simulink model "AuE6610_Project_EV"  (R2025a)
settings: Solver=FixedStepAuto  StartTime=0.0  StopTime=3353  FixedStep=1  RelTol=1e-3
values from neighbouring files (symbols this model uses):
  area_frontal = 2.18    [CV_Powertrain.m]    (also in EV_Powertrain.m; database.m)
  batt =     [battery_data.mat]
  curb_weight = 1377    [CV_Powertrain.m]    (also in EV_Powertrain.m; database.m)
  drag_coefficient = 0.29    [CV_Powertrain.m]    (also in EV_Powertrain.m; database.m)
  fdr = 4.21    [CV_Powertrain.m]    (also in EV_Powertrain.m; database.m)
  fdr_inertia = 0.02    [CV_Powertrain.m]    (also in EV_Powertrain.m; database.m)
  gear = [3.54, 1.91, 1.31, 0.97, 0.71, 0.62]    [CV_Powertrain.m]    (also in EV_Powertrain.m = 1.5; database.m)
  gear_no = [1, 2, 3, 4, 5, 6]    [CV_Powertrain.m]    (also in EV_Powertrain.m = 1; database.m = [1,2,3,4,5,6])
  mot =     [motor_data.mat]
  radius = 0.4318    [CV_Powertrain.m]    (also in EV_Powertrain.m; database.m)
  rho_air = 1.18    [CV_Powertrain.m]    (also in EV_Powertrain.m = 1.21; database.m)
  rolling_resistance_coefficient = 0.01    [CV_Powertrain.m]    (also in EV_Powertrain.m; database.m)
  trans_inertia = 0.04    [CV_Powertrain.m]    (also in EV_Powertrain.m; database.m)
  wheel_inertia = 0.95    [CV_Powertrain.m]    (also in EV_Powertrain.m; database.m)
libraries: slpidlib x2, simulink x2
settings Model: Creator=Qilun Zhu  LastModifiedBy=abhi
settings SolverCC: ZeroCrossAlgorithm=Adaptive  AlgebraicLoopSolver=TrustRegion
settings DataIOCC: ReturnWorkspaceOutputs=off
settings DebuggingCC: UnconnectedInputMsg=warning  UnconnectedOutputMsg=warning  UnconnectedLineMsg=warning  ArithmeticOperatorsInVariantConditions=warning
settings ModelReferenceCC: EnableRefExpFcnMdlSchedulingChecks=on
settings SFSimCC: SimUseLocalCustomCode=off  CustomCodeUndefinedFunction=UseInterfaceOnly
settings RTWCC: RTWUseLocalCustomCode=off  GPUComputeCapability=3.5  DLArmComputeVersion=19.05
settings CodeAppCC: StateflowObjectComments=on
settings SimscapeCC: SimscapeNormalizeSystem=off

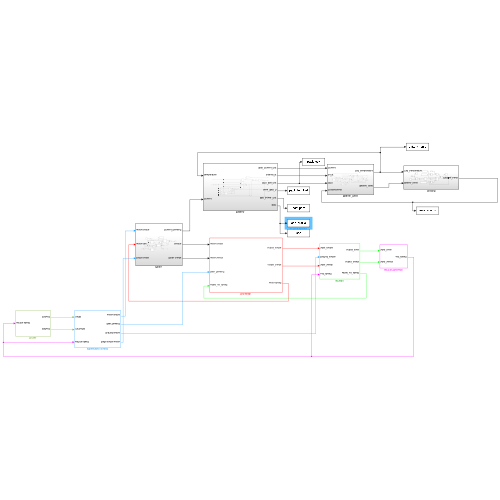
[thumbnail: Simulink's stored preview of the top-level diagram]
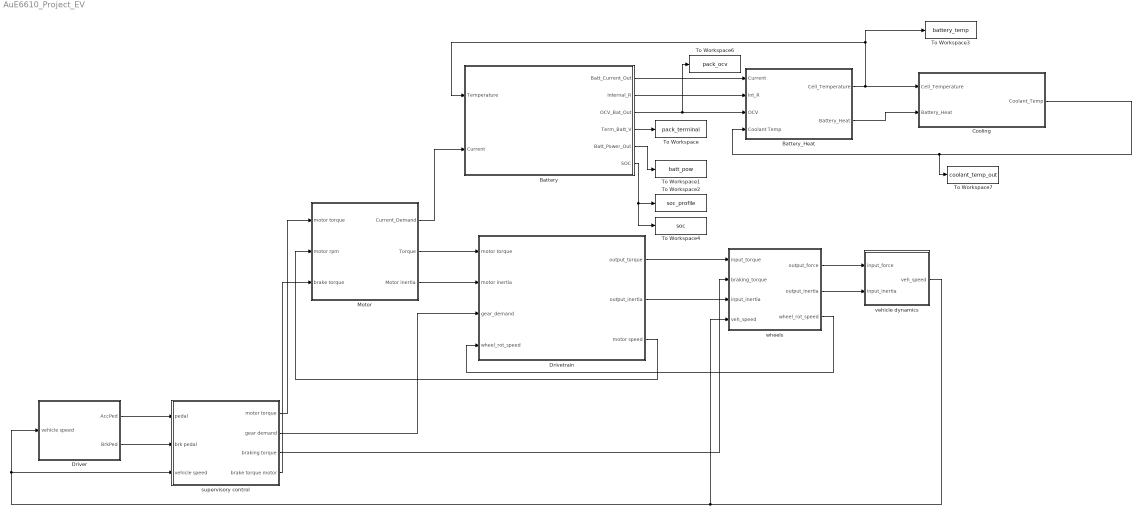
== system AuE6610_Project_EV ==
  Battery : Subsystem
  Battery_Heat : Subsystem
  Cooling : Subsystem
  Driver : Subsystem
  Drivetrain : Subsystem
  Motor : Subsystem
  To Workspace : ToWorkspace  VariableName=pack_terminal  SampleTime=-1
  To Workspace1 : ToWorkspace  VariableName=batt_pow  SampleTime=-1
  To Workspace2 : ToWorkspace  VariableName=soc_profile  SampleTime=300
  To Workspace3 : ToWorkspace  VariableName=battery_temp  SampleTime=-1
  To Workspace4 : ToWorkspace  VariableName=soc  SampleTime=-1
  To Workspace6 : ToWorkspace  VariableName=pack_ocv  SampleTime=-1
  To Workspace7 : ToWorkspace  VariableName=coolant_temp_out  SampleTime=-1
  supervisory control : Subsystem
  vehicle dynamics : Subsystem
  wheels : Subsystem
  wires:
  supervisory control/1(motor torque) -> Motor/1(motor torque)
  wheels/1(output_force) -> vehicle dynamics/1(input_force)
  wheels/2(output_inertia) -> vehicle dynamics/2(input_inertia)
  supervisory control/3(braking torque) -> wheels/2(braking_torque)
  Driver/1(AccPed) -> supervisory control/1(" pedal")
  supervisory control/2(gear demand) -> Drivetrain/3(gear_demand)
  Motor/2(Torque) -> Drivetrain/1(motor torque)
  Motor/3(Motor inertia) -> Drivetrain/2(motor inertia)
  wheels/3(wheel_rot_speed) -> Drivetrain/4(wheel_rot_speed)
  Drivetrain/1(output_torque) -> wheels/1(input_torque)
  Drivetrain/2(output_inertia) -> wheels/3(input_inertia)
  vehicle dynamics/1(veh_speed) -> Driver/1(vehicle speed), supervisory control/3(vehicle speed), wheels/4(veh_speed)
  Driver/2(BrkPed) -> supervisory control/2(" brk pedal")
  Motor/1(Current_Demand) -> Battery/2(Current)
  Battery_Heat/1(Cell_Temperature) -> Cooling/1(Cell_Temperature), To Workspace3/1, Battery/1(Temperature)
  Battery_Heat/2(Battery_Heat) -> Cooling/2(Battery_Heat)
  Cooling/1(Coolant_Temp) -> To Workspace7/1, Battery_Heat/4(Coolant Temp)
  Battery/3(OCV_Bat_Out) -> To Workspace6/1, Battery_Heat/3(OCV)
  Battery/2(Internal_R) -> Battery_Heat/2(Int_R)
  Battery/1(Batt_Current_Out) -> Battery_Heat/1(Current)
  Battery/4(Term_Batt_V) -> To Workspace/1
  Battery/5(Batt_Power_Out) -> To Workspace1/1
  Battery/6(SOC) -> To Workspace4/1, To Workspace2/1
  Drivetrain/3(motor speed) -> Motor/2(motor rpm)
  supervisory control/4(brake torque motor) -> Motor/3(brake torque)

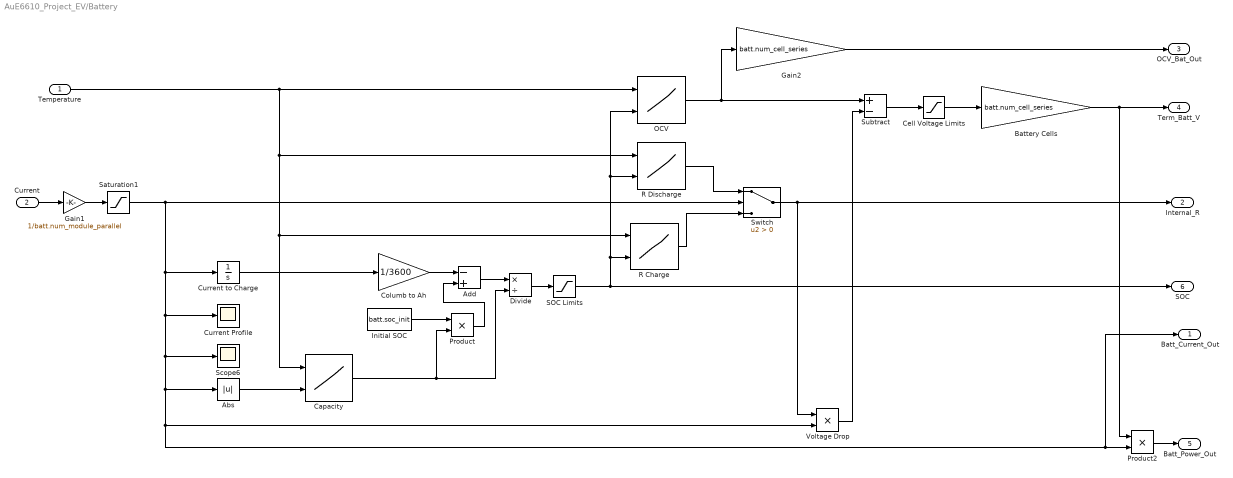
== system AuE6610_Project_EV/Battery ==
  Temperature : Inport
  Current : Inport  Port=2
  Abs : Abs  SaturateOnIntegerOverflow=off
  Add : Sum  Inputs=-+
  Battery Cells : Gain  Gain=batt.num_cell_series
  Capacity : Lookup_n-D  BreakpointsForDimension1=batt.cap_max.temp  BreakpointsForDimension2=batt.cap_max.curr  Table=batt.cap_max.cap_max  InternalRulePriority=Speed  RndMeth=Simplest
      settings: InputPortMap=u0,u1
  Cell Voltage Limits : Saturate  UpperLimit=batt.volt_max  LowerLimit=batt.volt_min
  Columb to Ah : Gain  Gain=1/3600
  Current Profile : Scope
      settings: ActiveDisplayYMinimum=-1  ActiveDisplayYMaximum=1
  Current to Charge : Integrator
  Divide : Product  Inputs=*/
  Gain1 : Gain  Gain=1/batt.num_module_parallel
  Gain2 : Gain  Gain=batt.num_cell_series
  Initial SOC : Constant  Value=batt.soc_init
  OCV : Lookup_n-D  BreakpointsForDimension1=batt.voc.temp  BreakpointsForDimension2=batt.voc.soc  Table=batt.voc.voc  InternalRulePriority=Speed  RndMeth=Simplest
      settings: InputPortMap=u0,u1
  Product : Product
  Product2 : Product
  R Charge : Lookup_n-D  BreakpointsForDimension1=batt.r_int_chg.temp  BreakpointsForDimension2=batt.r_int_chg.soc  Table=batt.r_int_chg.r_int  InternalRulePriority=Speed  RndMeth=Simplest
      settings: InputPortMap=u0,u1
  R Discharge : Lookup_n-D  BreakpointsForDimension1=batt.r_int_dis.temp  BreakpointsForDimension2=batt.r_int_dis.soc  Table=batt.r_int_dis.r_int  InternalRulePriority=Speed  RndMeth=Simplest
      settings: InputPortMap=u0,u1
  SOC Limits : Saturate  UpperLimit=batt.soc_max  LowerLimit=batt.soc_min
  Saturation1 : Saturate  UpperLimit=batt.curr_dis_max  LowerLimit=batt.curr_chg_max
  Scope6 : Scope
      settings: ActiveDisplayYMinimum=-1  ActiveDisplayYMaximum=1  DataLoggingVariableName=ScopeData7
  Subtract : Sum  Inputs=+-
  Switch : Switch  Criteria=u2 > Threshold  SaturateOnIntegerOverflow=off  InputSameDT=off
  Voltage Drop : Product
  Batt_Current_Out : Outport
  Internal_R : Outport  Port=2
  OCV_Bat_Out : Outport  Port=3
  Term_Batt_V : Outport  Port=4
  Batt_Power_Out : Outport  Port=5
  SOC : Outport  Port=6
  wires:
  Product2/1 -> Batt_Power_Out/1
  Subtract/1 -> Cell Voltage Limits/1
  Voltage Drop/1 -> Subtract/2
  Battery Cells/1 -> Term_Batt_V/1, Product2/1
  Gain2/1 -> OCV_Bat_Out/1
  R Charge/1 -> Switch/3
  R Discharge/1 -> Switch/1
  Temperature/1 -> Capacity/1, R Charge/1, R Discharge/1, OCV/1
  Divide/1 -> SOC Limits/1
  Add/1 -> Divide/1
  Cell Voltage Limits/1 -> Battery Cells/1
  Product/1 -> Add/2
  Switch/1 -> Internal_R/1, Voltage Drop/1
  Initial SOC/1 -> Product/1
  Abs/1 -> Capacity/2
  SOC Limits/1 -> R Charge/2, OCV/2, R Discharge/2, SOC/1
  Current/1 -> Gain1/1
  Current to Charge/1 -> Columb to Ah/1
  Columb to Ah/1 -> Add/1
  OCV/1 -> Gain2/1, Subtract/1
  Capacity/1 -> Product/2, Divide/2
  Saturation1/1 -> Batt_Current_Out/1, Product2/2, Voltage Drop/2, Abs/1, Scope6/1, Current Profile/1, Current to Charge/1, Switch/2
  Gain1/1 -> Saturation1/1

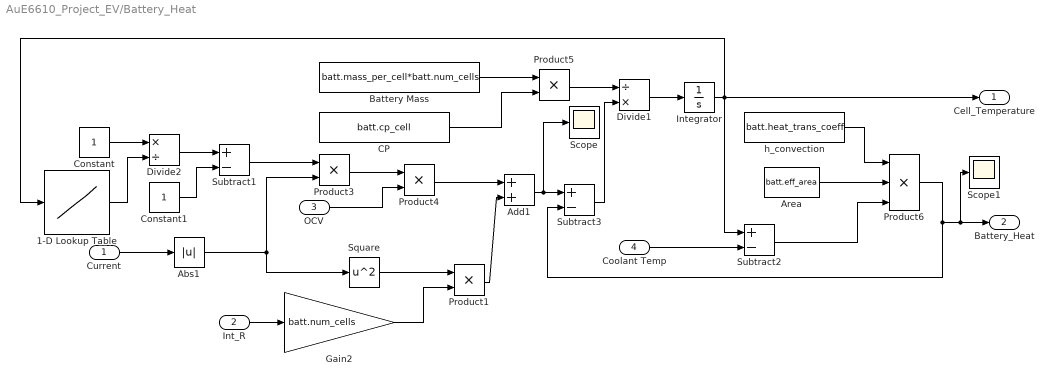
== system AuE6610_Project_EV/Battery_Heat ==
  Current : Inport
  Int_R : Inport  Port=2
  OCV : Inport  Port=3
  Coolant Temp : Inport  Port=4
  1-D Lookup Table : Lookup_n-D  NumberOfTableDimensions=1  BreakpointsForDimension1=batt.col_eff.temperature  Table=batt.col_eff.col_eff  InternalRulePriority=Speed  RndMeth=Simplest
  Abs1 : Abs  SaturateOnIntegerOverflow=off
  Add1 : Sum
  Area : Constant  Value=batt.eff_area
  Battery Mass : Constant  Value=batt.mass_per_cell*batt.num_cells
  CP : Constant  Value=batt.cp_cell
  Constant : Constant
  Constant1 : Constant
  Divide1 : Product  Inputs=/*
  Divide2 : Product  Inputs=*/
  Gain2 : Gain  Gain=batt.num_cells
  Integrator : Integrator  InitialCondition=25
  Product{1,3..5} (4 alike) : Product
  Product6 : Product  Inputs=3
  Scope : Scope
      settings: ActiveDisplayYMinimum=-1  ActiveDisplayYMaximum=1  DataLoggingVariableName=ScopeData2
  Scope1 : Scope
      settings: ActiveDisplayYMinimum=-470.32626460451758  ActiveDisplayYMaximum=4232.9363814406588  DataLoggingVariableName=ScopeData14
  Square : Math  Operator=square
  Subtract1 : Sum  Inputs=+-
  Subtract2 : Sum  Inputs=+-
  Subtract3 : Sum  Inputs=+-
  h_convection : Constant  Value=batt.heat_trans_coeff
  Cell_Temperature : Outport
  Battery_Heat : Outport  Port=2
  wires:
  Subtract2/1 -> Product6/3
  Area/1 -> Product6/2
  Subtract3/1 -> Divide1/2
  Battery Mass/1 -> Product5/1
  h_convection/1 -> Product6/1
  Add1/1 -> Scope/1, Subtract3/1
  Product4/1 -> Add1/1
  Product5/1 -> Divide1/1
  Gain2/1 -> Product1/2
  1-D Lookup Table/1 -> Divide2/2
  Subtract1/1 -> Product3/1
  Product6/1 -> Scope1/1, Battery_Heat/1, Subtract3/2
  OCV/1 -> Product4/2
  Divide1/1 -> Integrator/1
  Square/1 -> Product1/1
  Product3/1 -> Product4/1
  Divide2/1 -> Subtract1/1
  Constant/1 -> Divide2/1
  Int_R/1 -> Gain2/1
  Constant1/1 -> Subtract1/2
  Abs1/1 -> Square/1, Product3/2
  CP/1 -> Product5/2
  Integrator/1 -> Cell_Temperature/1, 1-D Lookup Table/1, Subtract2/1
  Coolant Temp/1 -> Subtract2/2
  Current/1 -> Abs1/1
  Product1/1 -> Add1/2

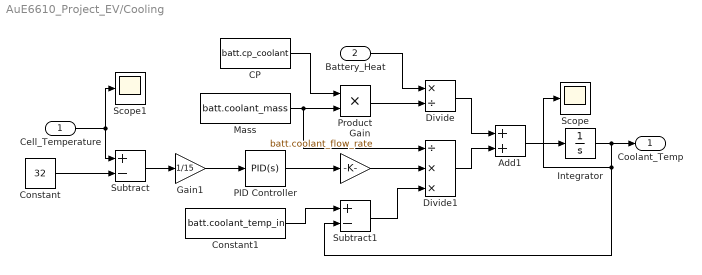
== system AuE6610_Project_EV/Cooling ==
  Cell_Temperature : Inport
  Battery_Heat : Inport  Port=2
  Add1 : Sum
  CP : Constant  Value=batt.cp_coolant
  Constant : Constant  Value=32
  Constant1 : Constant  Value=batt.coolant_temp_in
  Divide : Product  Inputs=*/
  Divide1 : Product  Inputs=/**
  Gain : Gain  Gain=batt.coolant_flow_rate
  Gain1 : Gain  Gain=1/15
  Integrator : Integrator  InitialCondition=25
  Mass : Constant  Value=batt.coolant_mass
  PID Controller : slpidlib/PID Controller  Controller=PID  Form=Parallel  TimeDomain=Continuous-time  UseExternalTs=off  SampleTime=-1  IntegratorMethod=Forward Euler  FilterMethod=Forward Euler  ControllerParametersSource=internal  P=1  I=0  UseKiTs=off  D=0  UseExternalDerivativeSource=off  N=100  UseFilter=on  TunerSelectOption=Transfer Function Based (PID Tuner App)  InitialConditionSource=internal  InitialConditionForIntegrator=0  InitialConditionForFilter=0  DifferentiatorICPrevScaledInput=0  ExternalReset=none  TrackingMode=off  Kt=1  LimitOutput=off  SatLimitsSource=internal  UpperSaturationLimit=inf  LowerSaturationLimit=-inf  LinearizeAsGain=on  AntiWindupMode=none  Kb=1  LimitIntegrator=off  UpperIntegratorSaturationLimit=inf  LowerIntegratorSaturationLimit=-inf  POutMin=[]  POutMax=[]  IOutMin=[]  IOutMax=[]  DOutMin=[]  DOutMax=[]  NOutMin=[]  NOutMax=[]  SumOutMin=[]  SumOutMax=[]  SaturationOutMin=[]  SaturationOutMax=[]  PParamMin=[]  PParamMax=[]  IParamMin=[]  IParamMax=[]  DParamMin=[]  DParamMax=[]  NParamMin=[]  NParamMax=[]  KbParamMin=[]  KbParamMax=[]  KtParamMin=[]  KtParamMax=[]  KbOutMin=[]  KbOutMax=[]  KtOutMin=[]  KtOutMax=[]  IntegratorOutMin=[]  IntegratorOutMax=[]  FilterOutMin=[]  FilterOutMax=[]  SumI1OutMin=[]  SumI1OutMax=[]  SumI2OutMin=[]  SumI2OutMax=[]  SumI3OutMin=[]  SumI3OutMax=[]  SumI4OutMin=[]  SumI4OutMax=[]  SumDOutMin=[]  SumDOutMax=[]  DifferentiatorOutMin=[]  DifferentiatorOutMax=[]  FilterDiffOutCoefMin=[]  FilterDiffOutCoefMax=[]  ReciprocalOutMin=[]  ReciprocalOutMax=[]  SumDenOutMin=[]  SumDenOutMax=[]  SumNumOutMin=[]  SumNumOutMax=[]  DivideOutMin=[]  DivideOutMax=[]  UdiffTsProdOutMin=[]  UdiffTsProdOutMax=[]  NTsProdOutMin=[]  NTsProdOutMax=[]  UintegralTsProdOutMin=[]  UintegralTsProdOutMax=[]  UngainTsProdOutMin=[]  UngainTsProdOutMax=[]  ClampingZeroOutDataTypeStr=Inherit: Inherit via back propagation  ClampingZeroOutMin=[]  ClampingZeroOutMax=[]  FilterDenConstantOutDataTypeStr=Inherit: Inherit via back propagation  FilterDenConstantOutMin=[]  FilterDenConstantOutMax=[]  PCopyOutDataTypeStr=Inherit: Inherit via back propagation  PCopyOutMin=[]  PCopyOutMax=[]  NCopyOutDataTypeStr=Inherit: Inherit via back propagation  NCopyOutMin=[]  NCopyOutMax=[]  IntegratorContinuousStateAttributes=''  IntegratorStateMustResolveToSignalObject=off  IntegratorRTWStateStorageClass=Auto  FilterContinuousStateAttributes=''  FilterStateMustResolveToSignalObject=off  FilterRTWStateStorageClass=Auto  ParallelPVariant=InternalParameters  IdealPVariant=Disabled  IVariant=InternalParameters  DVariant=InternalParameters  IntegratorVariant=Continuous  SatVariant=Disabled  AWVariant=Passthrough  PCopyVariant=Disabled  TRVariant=Disabled  FdbkBlocksVariant=Forward  IdealPFdbkVariant=Disabled  SatFdbkVariant=Disabled  DerivativeFilterVariant=ContFilter  NVariant=InternalParameters  NCopyVariant=Disabled  FilterICVariant=InternalICsFilter  IntegratorICVariant=InternalICs  ExternalResetVariant=Disabled  TRSumVariant=Passthrough  SumFdbkVariant=Disabled  SumVariant=Sum_PID  TsampFilterVariant=InternalTs  TsampNgainVariant=Passthrough  TsampIntegralVariant=Disabled_SignalSpec  ExternalSaturationOutDataTypeStr=Inherit: Same as second input  DerivativeSourceVariant=ErrorSignal  PreIntVariant=InternalPreInt
  Product : Product
  Scope : Scope
      settings: ActiveDisplayYMinimum=24.835198130319185  ActiveDisplayYMaximum=26.483216827127347  DataLoggingVariableName=ScopeData9
  Scope1 : Scope
      settings: ActiveDisplayYMinimum=23.800501733675897  ActiveDisplayYMaximum=35.795484396916919  DataLoggingVariableName=ScopeData15
  Subtract : Sum  Inputs=+-
  Subtract1 : Sum  Inputs=+-
  Coolant_Temp : Outport
  wires:
  Integrator/1 -> Scope/1, Subtract1/2, Coolant_Temp/1
  Add1/1 -> Integrator/1
  Divide1/1 -> Add1/2
  Product/1 -> Divide/2
  PID Controller/1 -> Gain/1
  Constant1/1 -> Subtract1/1
  Subtract1/1 -> Divide1/3
  Constant/1 -> Subtract/2
  Mass/1 -> Product/2, Divide1/1
  CP/1 -> Product/1
  Divide/1 -> Add1/1
  Cell_Temperature/1 -> Scope1/1, Subtract/1
  Gain/1 -> Divide1/2
  Battery_Heat/1 -> Divide/1
  Subtract/1 -> Gain1/1
  Gain1/1 -> PID Controller/1

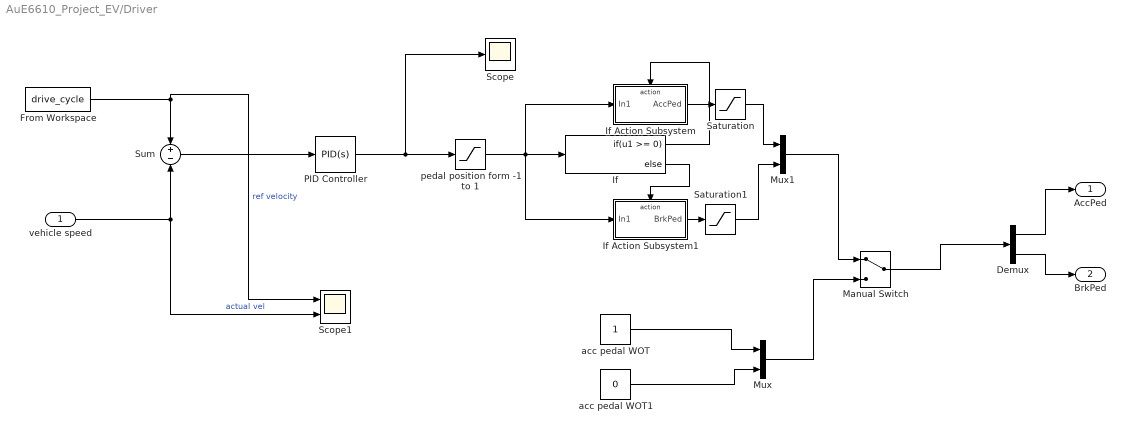
== system AuE6610_Project_EV/Driver ==
  vehicle speed : Inport
  Demux : Demux  Outputs=2
  From Workspace : FromWorkspace  VariableName=drive_cycle
  If : If  IfExpression=u1 >= 0
  If Action Subsystem : Subsystem  TreatAsAtomicUnit=on
  If Action Subsystem1 : Subsystem  TreatAsAtomicUnit=on
  Manual Switch : ManualSwitch
  Mux : Mux  Inputs=2
  Mux1 : Mux  Inputs=2
  PID Controller : slpidlib/PID Controller  Controller=PID  Form=Parallel  TimeDomain=Continuous-time  UseExternalTs=off  SampleTime=-1  IntegratorMethod=Forward Euler  FilterMethod=Forward Euler  ControllerParametersSource=internal  P=0.2  I=0.2  UseKiTs=off  D=0  UseExternalDerivativeSource=off  N=10  UseFilter=on  TunerSelectOption=Transfer Function Based (PID Tuner App)  InitialConditionSource=internal  InitialConditionForIntegrator=0  InitialConditionForFilter=0  DifferentiatorICPrevScaledInput=0  ExternalReset=none  TrackingMode=off  Kt=1  LimitOutput=off  SatLimitsSource=internal  UpperSaturationLimit=inf  LowerSaturationLimit=-inf  LinearizeAsGain=on  AntiWindupMode=none  Kb=1  LimitIntegrator=off  UpperIntegratorSaturationLimit=inf  LowerIntegratorSaturationLimit=-inf  POutMin=[]  POutMax=[]  IOutMin=[]  IOutMax=[]  DOutMin=[]  DOutMax=[]  NOutMin=[]  NOutMax=[]  SumOutMin=[]  SumOutMax=[]  SaturationOutMin=[]  SaturationOutMax=[]  PParamMin=[]  PParamMax=[]  IParamMin=[]  IParamMax=[]  DParamMin=[]  DParamMax=[]  NParamMin=[]  NParamMax=[]  KbParamMin=[]  KbParamMax=[]  KtParamMin=[]  KtParamMax=[]  KbOutMin=[]  KbOutMax=[]  KtOutMin=[]  KtOutMax=[]  IntegratorOutMin=[]  IntegratorOutMax=[]  FilterOutMin=[]  FilterOutMax=[]  SumI1OutMin=[]  SumI1OutMax=[]  SumI2OutMin=[]  SumI2OutMax=[]  SumI3OutMin=[]  SumI3OutMax=[]  SumI4OutMin=[]  SumI4OutMax=[]  SumDOutMin=[]  SumDOutMax=[]  DifferentiatorOutMin=[]  DifferentiatorOutMax=[]  FilterDiffOutCoefMin=[]  FilterDiffOutCoefMax=[]  ReciprocalOutMin=[]  ReciprocalOutMax=[]  SumDenOutMin=[]  SumDenOutMax=[]  SumNumOutMin=[]  SumNumOutMax=[]  DivideOutMin=[]  DivideOutMax=[]  UdiffTsProdOutMin=[]  UdiffTsProdOutMax=[]  NTsProdOutMin=[]  NTsProdOutMax=[]  UintegralTsProdOutMin=[]  UintegralTsProdOutMax=[]  UngainTsProdOutMin=[]  UngainTsProdOutMax=[]  ClampingZeroOutDataTypeStr=Inherit: Inherit via back propagation  ClampingZeroOutMin=[]  ClampingZeroOutMax=[]  FilterDenConstantOutDataTypeStr=Inherit: Inherit via back propagation  FilterDenConstantOutMin=[]  FilterDenConstantOutMax=[]  PCopyOutDataTypeStr=Inherit: Inherit via back propagation  PCopyOutMin=[]  PCopyOutMax=[]  NCopyOutDataTypeStr=Inherit: Inherit via back propagation  NCopyOutMin=[]  NCopyOutMax=[]  IntegratorContinuousStateAttributes=''  IntegratorStateMustResolveToSignalObject=off  IntegratorRTWStateStorageClass=Auto  FilterContinuousStateAttributes=''  FilterStateMustResolveToSignalObject=off  FilterRTWStateStorageClass=Auto  ParallelPVariant=InternalParameters  IdealPVariant=Disabled  IVariant=InternalParameters  DVariant=InternalParameters  IntegratorVariant=Continuous  SatVariant=Disabled  AWVariant=Passthrough  PCopyVariant=Disabled  TRVariant=Disabled  FdbkBlocksVariant=Forward  IdealPFdbkVariant=Disabled  SatFdbkVariant=Disabled  DerivativeFilterVariant=ContFilter  NVariant=InternalParameters  NCopyVariant=Disabled  FilterICVariant=InternalICsFilter  IntegratorICVariant=InternalICs  ExternalResetVariant=Disabled  TRSumVariant=Passthrough  SumFdbkVariant=Disabled  SumVariant=Sum_PID  TsampFilterVariant=InternalTs  TsampNgainVariant=Passthrough  TsampIntegralVariant=Disabled_SignalSpec  ExternalSaturationOutDataTypeStr=Inherit: Same as second input  DerivativeSourceVariant=ErrorSignal  PreIntVariant=InternalPreInt
  Saturation : Saturate  UpperLimit=1  LowerLimit=0
  Saturation1 : Saturate  UpperLimit=0  LowerLimit=-1
  Scope : Scope
      settings: ActiveDisplayYMinimum=-1  ActiveDisplayYMaximum=1  DataLoggingVariableName=ScopeData8
  Scope1 : Scope  NumInputPorts=2
      settings: ActiveDisplayYMinimum=4.7265051109155625  ActiveDisplayYMaximum=36.463746846467487
  Sum : Sum  Inputs=+-
  acc pedal WOT : Constant
  acc pedal WOT1 : Constant  Value=0
  pedal position form -1 to 1 : Saturate  UpperLimit=1  LowerLimit=-1  ZeroCross=off
  AccPed : Outport
  BrkPed : Outport  Port=2
  wires:
  Manual Switch/1 -> Demux/1
  If/1 -> If Action Subsystem/Action
  If/2 -> If Action Subsystem1/Action
  Sum/1 -> PID Controller/1
  pedal position form -1 to 1/1 -> If/1, If Action Subsystem1/1(In1), If Action Subsystem/1(In1)
  acc pedal WOT/1 -> Mux/1
  acc pedal WOT1/1 -> Mux/2
  Mux/1 -> Manual Switch/2
  Demux/1 -> AccPed/1
  Demux/2 -> BrkPed/1
  Mux1/1 -> Manual Switch/1
  From Workspace/1 -> Scope1/1, Sum/1  "ref velocity"
  vehicle speed/1 -> Scope1/2, Sum/2  "actual vel"
  PID Controller/1 -> Scope/1, pedal position form -1 to 1/1
  If Action Subsystem/1(AccPed) -> Saturation/1
  Saturation/1 -> Mux1/1
  If Action Subsystem1/1(BrkPed) -> Saturation1/1
  Saturation1/1 -> Mux1/2

== system AuE6610_Project_EV/Drivetrain ==
  motor torque : Inport
  motor inertia : Inport  Port=2
  gear_demand : Inport  Port=3
  wheel_rot_speed : Inport  Port=4
  Scope : Scope
      settings: ActiveDisplayYMinimum=-2734.288443170964  ActiveDisplayYMaximum=2734.288443170964  DataLoggingVariableName=ScopeData4
  Scope1 : Scope
      settings: ActiveDisplayYMinimum=-1  ActiveDisplayYMaximum=1  DataLoggingVariableName=ScopeData6
  final drive : Subsystem
  transmission : Subsystem
  output_torque : Outport
  output_inertia : Outport  Port=2
  motor speed : Outport  Port=3
  wires:
  transmission/3(motor_speed) -> motor speed/1
  transmission/2(output_inertia) -> final drive/2(input_inertia)
  transmission/1(output_torque) -> Scope1/1, final drive/1(input_torque)
  motor inertia/1 -> transmission/3(input_inertia)
  final drive/3(trans_speed) -> transmission/4(trans_speed)
  motor torque/1 -> transmission/2(input_torque)
  gear_demand/1 -> transmission/1(gear_demand)
  final drive/1(output_torque) -> Scope/1, output_torque/1
  wheel_rot_speed/1 -> final drive/3(wheel_rot_speed)
  final drive/2(output_inertia) -> output_inertia/1

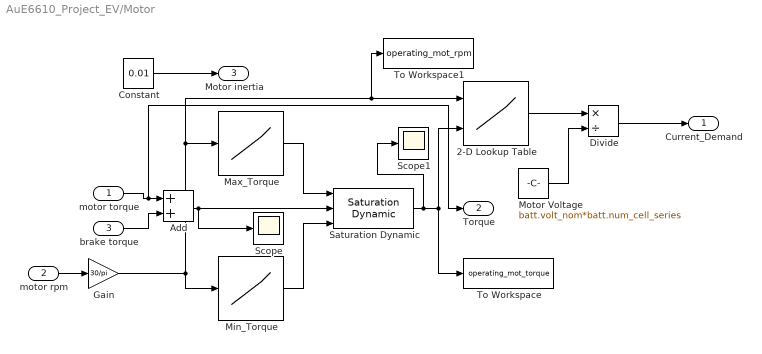
== system AuE6610_Project_EV/Motor ==
  motor torque : Inport
  motor rpm : Inport  Port=2
  brake torque : Inport  Port=3
  2-D Lookup Table : Lookup_n-D  BreakpointsForDimension1=mot.efficiency.RPM  BreakpointsForDimension2=mot.efficiency.Torque  Table=mot.efficiency.elec_power  InternalRulePriority=Speed  RndMeth=Simplest
      settings: InputPortMap=u0,u1
  Add : Sum
  Constant : Constant  Value=0.01
  Divide : Product  Inputs=*/
  Gain : Gain  Gain=30/pi
  Max_Torque : Lookup_n-D  NumberOfTableDimensions=1  BreakpointsForDimension1=mot.max_torque.RPM  Table=mot.max_torque.Torque  InternalRulePriority=Speed  RndMeth=Simplest
  Min_Torque : Lookup_n-D  NumberOfTableDimensions=1  BreakpointsForDimension1=mot.min_torque.RPM  Table=mot.min_torque.Torque  InternalRulePriority=Speed  RndMeth=Simplest
  Motor Voltage : Constant  Value=batt.volt_nom*batt.num_cell_series
  Saturation Dynamic : simulink/Discontinuities/Saturation Dynamic  OutMin=[]  OutMax=[]  OutDataTypeStr=Inherit: Same as second input  OutDataType=fixdt(1, 16)  OutScaling=2^-10  DoSatur=off
  Scope : Scope
      settings: ActiveDisplayYMinimum=-690.21630100474192  ActiveDisplayYMaximum=1537.1191137749931
  Scope1 : Scope
      settings: ActiveDisplayYMinimum=-405.92168099331411  ActiveDisplayYMaximum=405.92168099331411  DataLoggingVariableName=ScopeData3
  To Workspace : ToWorkspace  VariableName=operating_mot_torque  SampleTime=-1
  To Workspace1 : ToWorkspace  VariableName=operating_mot_rpm  SampleTime=-1
  Current_Demand : Outport
  Torque : Outport  Port=2
  Motor inertia : Outport  Port=3
  wires:
  Saturation Dynamic/1 -> Scope1/1, To Workspace/1, 2-D Lookup Table/2
  Min_Torque/1 -> Saturation Dynamic/3
  Constant/1 -> Motor inertia/1
  Max_Torque/1 -> Saturation Dynamic/1
  motor rpm/1 -> Gain/1
  2-D Lookup Table/1 -> Divide/1
  Divide/1 -> Current_Demand/1
  Motor Voltage/1 -> Divide/2
  Gain/1 -> Max_Torque/1, To Workspace1/1, 2-D Lookup Table/1, Min_Torque/1
  motor torque/1 -> Torque/1, Add/1
  brake torque/1 -> Add/2
  Add/1 -> Scope/1, Saturation Dynamic/2

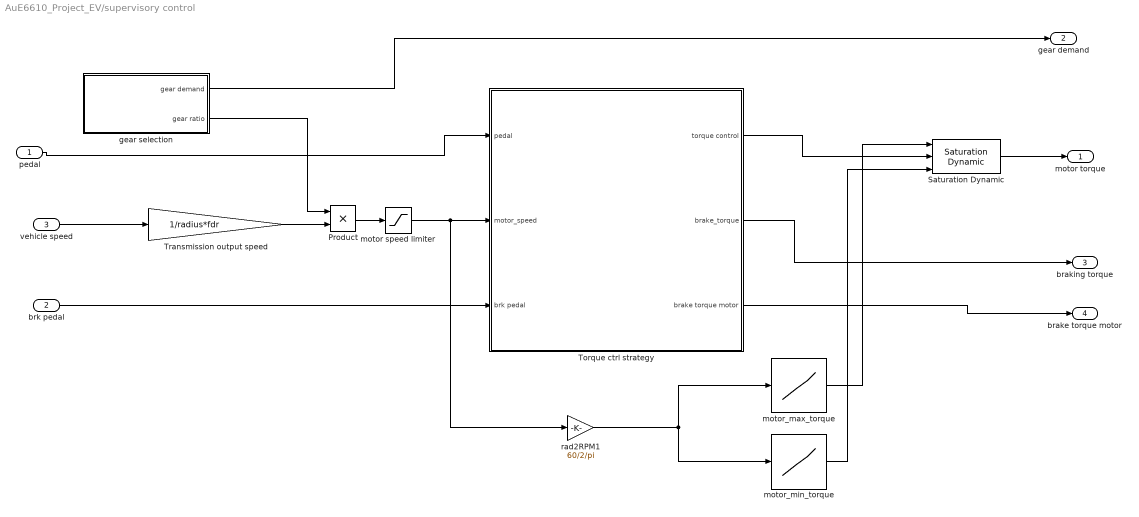
== system AuE6610_Project_EV/supervisory control ==
  " pedal" : Inport
  " brk pedal" : Inport  Port=2
  vehicle speed : Inport  Port=3
  Product : Product
  Saturation Dynamic : simulink/Discontinuities/Saturation Dynamic  OutMin=[]  OutMax=[]  OutDataTypeStr=Inherit: Same as second input  OutDataType=fixdt(1, 16)  OutScaling=2^-10  DoSatur=off
  Torque ctrl strategy : Subsystem
  Transmission output speed : Gain  Gain=1/radius*fdr
  gear selection : Subsystem
  motor speed limiter : Saturate  UpperLimit=6800/60*2*pi  LowerLimit=500/60*2*pi
  motor_max_torque : Lookup_n-D  NumberOfTableDimensions=1  BreakpointsForDimension1=mot.max_torque.RPM  Table=mot.max_torque.Torque  InternalRulePriority=Speed  RndMeth=Simplest
  motor_min_torque : Lookup_n-D  NumberOfTableDimensions=1  BreakpointsForDimension1=mot.min_torque.RPM  Table=mot.min_torque.Torque  InternalRulePriority=Speed  RndMeth=Simplest
  rad2RPM1 : Gain  Gain=60/2/pi
  motor torque : Outport
  gear demand : Outport  Port=2
  braking torque : Outport  Port=3
  brake torque motor : Outport  Port=4
  wires:
  motor_max_torque/1 -> Saturation Dynamic/1
  motor_min_torque/1 -> Saturation Dynamic/3
  Torque ctrl strategy/1(torque control) -> Saturation Dynamic/2
  Saturation Dynamic/1 -> motor torque/1
  rad2RPM1/1 -> motor_max_torque/1, motor_min_torque/1
  motor speed limiter/1 -> rad2RPM1/1, Torque ctrl strategy/2(motor_speed)
  Product/1 -> motor speed limiter/1
  " pedal"/1 -> Torque ctrl strategy/1(pedal)
  vehicle speed/1 -> Transmission output speed/1
  gear selection/2(gear ratio) -> Product/1
  Transmission output speed/1 -> Product/2
  gear selection/1(gear demand) -> gear demand/1
  " brk pedal"/1 -> Torque ctrl strategy/3(" brk pedal")
  Torque ctrl strategy/2(brake_torque) -> braking torque/1
  Torque ctrl strategy/3(brake torque motor) -> brake torque motor/1

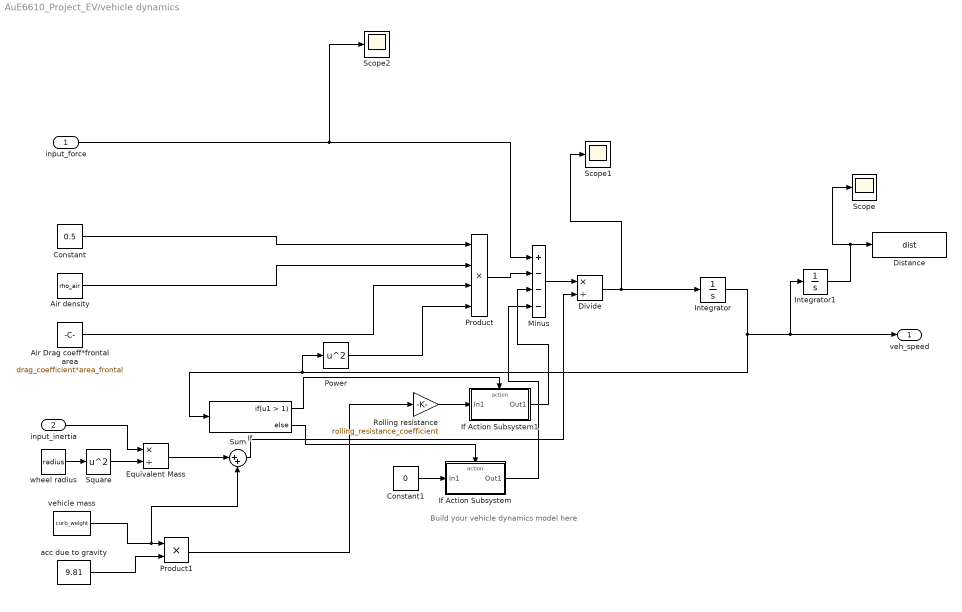
== system AuE6610_Project_EV/vehicle dynamics ==
  note: Build your vehicle dynamics model here
  input_force : Inport
  input_inertia : Inport  Port=2
  Air Drag coeff*frontal area : Constant  Value=drag_coefficient*area_frontal
  Air density : Constant  Value=rho_air
  Constant : Constant  Value=0.5
  Constant1 : Constant  Value=0
  Distance : ToWorkspace  VariableName=dist  SampleTime=-1
      settings: Save2DSignal=2-D array (concatenate along first dimension)
  Divide : Product  Inputs=*/
  Equivalent Mass : Product  Inputs=*/
  If : If  IfExpression=u1 > 1
  If Action Subsystem : Subsystem  TreatAsAtomicUnit=on
  If Action Subsystem1 : Subsystem  TreatAsAtomicUnit=on
  Integrator : Integrator
  Integrator1 : Integrator
  Minus : Sum  Inputs=+---
  Power : Math  Operator=square
  Product : Product  Inputs=4
  Product1 : Product
  "Rolling resistance " : Gain  Gain=rolling_resistance_coefficient
  Scope : Scope
      settings: ActiveDisplayYMinimum=-2221.2760263403779  ActiveDisplayYMaximum=19991.484237063407  DataLoggingVariableName=ScopeData5
  Scope1 : Scope
      settings: ActiveDisplayYMinimum=-1.1974689973392995E+78  ActiveDisplayYMaximum=1.330521108154777E+77  DataLoggingVariableName=ScopeData10
  Scope2 : Scope
      settings: ActiveDisplayYMinimum=-11552.03203293719  ActiveDisplayYMaximum=6560.4782964346941  DataLoggingVariableName=ScopeData11
  Square : Math  Operator=square
  Sum : Sum  Inputs=|++
  acc due to gravity : Constant  Value=9.81
  vehicle mass : Constant  Value=curb_weight
  wheel radius : Constant  Value=radius
  veh_speed : Outport
  wires:
  Product/1 -> Minus/2
  Integrator/1 -> If/1, Power/1, Integrator1/1, veh_speed/1
  If/1 -> If Action Subsystem1/Action
  If Action Subsystem1/1(Out1) -> Minus/3
  Divide/1 -> Scope1/1, Integrator/1
  If Action Subsystem/1(Out1) -> Minus/4
  Minus/1 -> Divide/1
  "Rolling resistance "/1 -> If Action Subsystem1/1(In1)
  If/2 -> If Action Subsystem/Action
  input_force/1 -> Scope2/1, Minus/1
  Constant/1 -> Product/1
  Air density/1 -> Product/2
  Air Drag coeff*frontal area/1 -> Product/3
  Power/1 -> Product/4
  vehicle mass/1 -> Sum/2, Product1/1
  acc due to gravity/1 -> Product1/2
  Product1/1 -> "Rolling resistance "/1
  Constant1/1 -> If Action Subsystem/1(In1)
  wheel radius/1 -> Square/1
  Square/1 -> Equivalent Mass/2
  input_inertia/1 -> Equivalent Mass/1
  Equivalent Mass/1 -> Sum/1
  Sum/1 -> Divide/2
  Integrator1/1 -> Scope/1, Distance/1

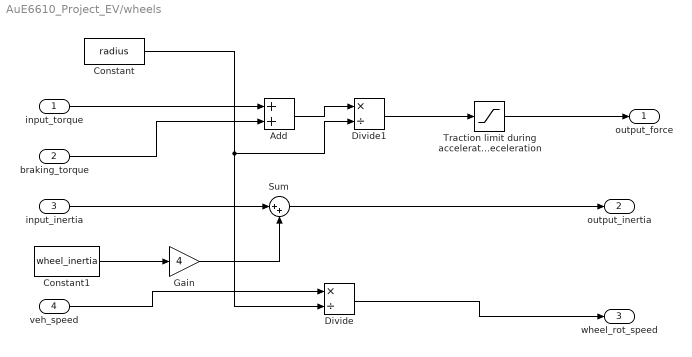
== system AuE6610_Project_EV/wheels ==
  input_torque : Inport
  braking_torque : Inport  Port=2
  input_inertia : Inport  Port=3
  veh_speed : Inport  Port=4
  Add : Sum
  Constant : Constant  Value=radius
  Constant1 : Constant  Value=wheel_inertia
  Divide : Product  Inputs=*/
  Divide1 : Product  Inputs=*/
  Gain : Gain  Gain=4
  Sum : Sum  Inputs=|++
  Traction limit during acceleration or deceleration : Saturate  UpperLimit=9740.781  LowerLimit=-9740.781
  output_force : Outport
  output_inertia : Outport  Port=2
  wheel_rot_speed : Outport  Port=3
  wires:
  Traction limit during acceleration or deceleration/1 -> output_force/1
  Constant/1 -> Divide1/2, Divide/2
  veh_speed/1 -> Divide/1
  Divide/1 -> wheel_rot_speed/1
  Constant1/1 -> Gain/1
  input_inertia/1 -> Sum/1
  Gain/1 -> Sum/2
  Sum/1 -> output_inertia/1
  input_torque/1 -> Add/1
  braking_torque/1 -> Add/2
  Add/1 -> Divide1/1
  Divide1/1 -> Traction limit during acceleration or deceleration/1

== system AuE6610_Project_EV/Driver/If Action Subsystem ==
  In1 : Inport
  Action Port : ActionPort  ActionPortLabel=if(u1 >= 0)
  AccPed : Outport
  wires:
  In1/1 -> AccPed/1

== system AuE6610_Project_EV/Driver/If Action Subsystem1 ==
  In1 : Inport
  Action Port : ActionPort  ActionPortLabel=else
  BrkPed : Outport
  wires:
  In1/1 -> BrkPed/1

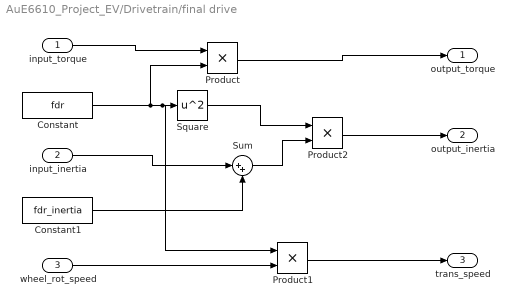
== system AuE6610_Project_EV/Drivetrain/final drive ==
  input_torque : Inport
  input_inertia : Inport  Port=2
  wheel_rot_speed : Inport  Port=3
  Constant : Constant  Value=fdr
  Constant1 : Constant  Value=fdr_inertia
  Product : Product
  Product1 : Product
  Product2 : Product
  Square : Math  Operator=square
  Sum : Sum  Inputs=|++
  output_torque : Outport
  output_inertia : Outport  Port=2
  trans_speed : Outport  Port=3
  wires:
  input_torque/1 -> Product/1
  Constant/1 -> Square/1, Product1/1, Product/2
  Product/1 -> output_torque/1
  input_inertia/1 -> Sum/1
  Constant1/1 -> Sum/2
  wheel_rot_speed/1 -> Product1/2
  Product1/1 -> trans_speed/1
  Product2/1 -> output_inertia/1
  Sum/1 -> Product2/2
  Square/1 -> Product2/1

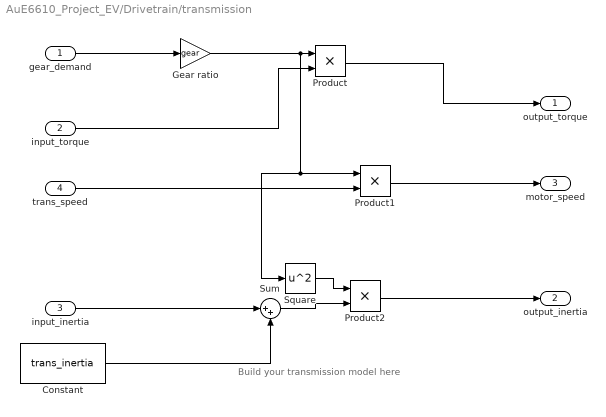
== system AuE6610_Project_EV/Drivetrain/transmission ==
  note: Build your transmission model here
  gear_demand : Inport
  input_torque : Inport  Port=2
  input_inertia : Inport  Port=3
  trans_speed : Inport  Port=4
  Constant : Constant  Value=trans_inertia
  Gear ratio : Gain  Gain=gear
  Product : Product
  Product1 : Product
  Product2 : Product
  Square : Math  Operator=square
  Sum : Sum  Inputs=|++
  output_torque : Outport
  output_inertia : Outport  Port=2
  motor_speed : Outport  Port=3
  wires:
  gear_demand/1 -> Gear ratio/1
  Gear ratio/1 -> Product1/1, Square/1, Product/1
  input_torque/1 -> Product/2
  Product/1 -> output_torque/1
  Constant/1 -> Sum/2
  input_inertia/1 -> Sum/1
  trans_speed/1 -> Product1/2
  Product1/1 -> motor_speed/1
  Square/1 -> Product2/1
  Sum/1 -> Product2/2
  Product2/1 -> output_inertia/1

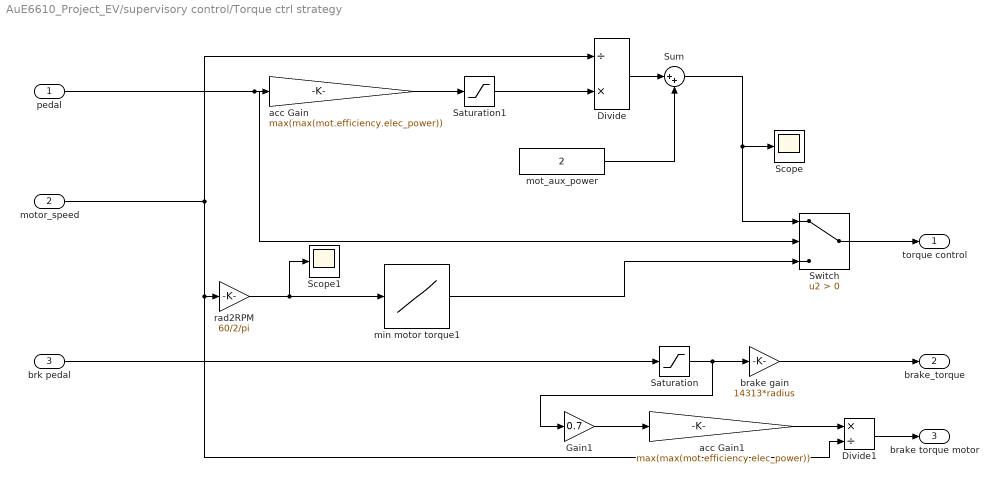
== system AuE6610_Project_EV/supervisory control/Torque ctrl strategy ==
  pedal : Inport
  motor_speed : Inport  Port=2
  " brk pedal" : Inport  Port=3
  Divide : Product  Inputs=/*
  Divide1 : Product  Inputs=*/
  Gain1 : Gain  Gain=0.7
  Saturation : Saturate  UpperLimit=0  LowerLimit=-1
  Saturation1 : Saturate  UpperLimit=max(max(mot.efficiency.elec_power))  LowerLimit=0  ZeroCross=off
  Scope : Scope
      settings: ActiveDisplayYMinimum=-399.84906412460754  ActiveDisplayYMaximum=4052.1828052874889  DataLoggingVariableName=ScopeData12
  Scope1 : Scope
      settings: ActiveDisplayYMinimum=400.00000000000006  ActiveDisplayYMaximum=600  DataLoggingVariableName=ScopeData13
  Sum : Sum  Inputs=|++
  Switch : Switch  Criteria=u2 > Threshold  ZeroCross=off  SaturateOnIntegerOverflow=off  InputSameDT=off
  acc Gain : Gain  Gain=max(max(mot.efficiency.elec_power))
  acc Gain1 : Gain  Gain=max(max(mot.efficiency.elec_power))
  brake gain : Gain  Gain=14313*radius
  min motor torque1 : Lookup_n-D  NumberOfTableDimensions=1  BreakpointsForDimension1=mot.min_torque.RPM  Table=mot.min_torque.Torque  InternalRulePriority=Speed  RndMeth=Simplest
  mot_aux_power : Constant  Value=2
  rad2RPM : Gain  Gain=60/2/pi
  torque control : Outport
  brake_torque : Outport  Port=2
  brake torque motor : Outport  Port=3
  wires:
  min motor torque1/1 -> Switch/3
  Switch/1 -> torque control/1
  brake gain/1 -> brake_torque/1
  Saturation/1 -> Gain1/1, brake gain/1
  pedal/1 -> Switch/2, acc Gain/1
  Saturation1/1 -> Divide/2
  motor_speed/1 -> Divide1/2, rad2RPM/1, Divide/1
  Divide/1 -> Sum/1
  mot_aux_power/1 -> Sum/2
  acc Gain/1 -> Saturation1/1
  Sum/1 -> Scope/1, Switch/1
  rad2RPM/1 -> Scope1/1, min motor torque1/1
  " brk pedal"/1 -> Saturation/1
  Gain1/1 -> acc Gain1/1
  acc Gain1/1 -> Divide1/1
  Divide1/1 -> brake torque motor/1

== system AuE6610_Project_EV/supervisory control/gear selection ==
  Constant : Constant  Value=gear
  Constant1 : Constant  Value=gear_no
  gear demand : Outport
  gear ratio : Outport  Port=2
  wires:
  Constant1/1 -> gear demand/1
  Constant/1 -> gear ratio/1

== system AuE6610_Project_EV/vehicle dynamics/If Action Subsystem ==
  In1 : Inport
  Action Port : ActionPort  ActionPortLabel=else
  Out1 : Outport
  wires:
  In1/1 -> Out1/1

== system AuE6610_Project_EV/vehicle dynamics/If Action Subsystem1 ==
  In1 : Inport
  Action Port : ActionPort  ActionPortLabel=if(u1 > 1)
  Out1 : Outport
  wires:
  In1/1 -> Out1/1
